simulink model "stm32f0_iap_boot"  (Simulink 7.3)
settings: Solver=ode3  SolverMode=SingleTasking  StartTime=0.0  StopTime=10.0  RelTol=1e-3
PreLoadFcn:
  | waijung.modelPreload; % Required for working with Waijung Blockset. Do not remove.
undefined symbols (not defined in the file): LQFP48, STM32F072CB
libraries: simulink x14, stm32f0_flash_lib x10, stm32f0_boot_lib x3, waijung_crc_lib x3, stm32f0_io_lib x1, stm32f0_reset_lib x1, stm32f0_device_config_lib x1
CloseFcn:
  | waijung.modelClose; % Required for working with Waijung Blockset. Do not remove.
settings Model: Creator=Nav  LastModifiedBy=Krisada
settings OptimizationCC: OptimizeModelRefInitCode=on  LifeSpan=1
settings HardwareCC: ProdEndianess=LittleEndian  ProdHWDeviceType=ARM Compatible->Cortex - M0  TargetEndianess=LittleEndian  TargetHWDeviceType=ARM Compatible->Cortex - M0
settings RTWCC: SystemTargetFile=stm32f0.tlc  GenerateMakefile=off  TemplateMakefile=ert_default_tmf  Description=STM32F0 Target  ProcessScript=stm32f0_make_rtw_hook
settings CodeAppCC: IgnoreCustomStorageClasses=off
settings STFCustomTargetCC: ModelReferenceCompliant=off  CombineOutputUpdateFcns=on  ERTCustomFileBanners=on  SupportContinuousTime=off  SupportNonInlinedSFcns=off  SystemTargetFile=stm32f0.tlc
settings ERTTargetCC: MultiwordLength=2048  ModelReferenceCompliant=off  ParMdlRefBuildCompliant=off  CompOptLevelCompliant=off  ERTFirstTimeCompliant=off  ModelStepFunctionPrototypeControlCompliant=off  CPPClassGenCompliant=off  InlinedParameterPlacement=NonHierarchical  ERTSrcFileBannerTemplate=stm32f0_code_template.cgt  ERTHdrFileBannerTemplate=stm32f0_code_template.cgt  ERTDataSrcFileTemplate=stm32f0_code_template.cgt  ERTDataHdrFileTemplate=stm32f0_code_template.cgt  ERTCustomFileTemplate=stm32f0_file_process.tlc

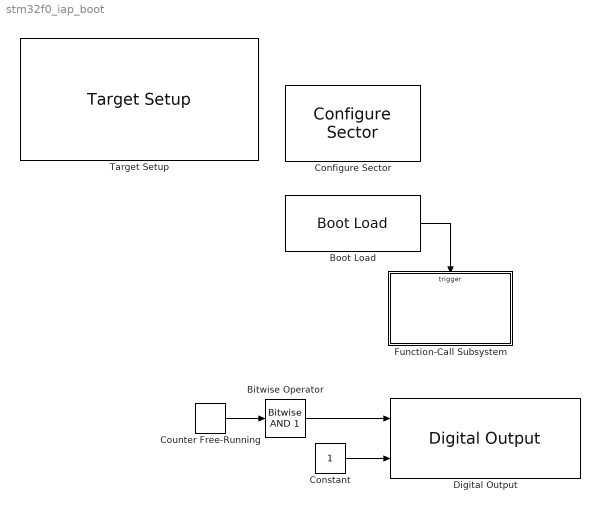
== system stm32f0_iap_boot ==
  Bitwise Operator : simulink/Logic and Bit Operations/Bitwise Operator  logicop=AND  UseBitMask=on  BitMask=1  BitMaskRealWorld=Stored Integer
  Boot Load : stm32f0_boot_lib/Boot Load  conf=Boot  flashorigin=0x8000000  flashlength=0x100000  enableisr=on  usersector=Sector 9: 0x080A0000 - 0x080BFFFF  sampletime=-1  sampletimestr=0.1  blockid=BootLoad  inputarray=[]  inputlabelarray={}  outputarray=[7]  outputlabelarray={'Call ISR'}  compat=0  confstr="[\"80A0000\",\"9\",\"8000000\"]"
  Configure Sector : stm32f0_boot_lib/Configure Sector  conf=Configure  flashorigin=0x8000000  flashlength=0x004000  enableisr=off  usersector=Sector 5: 0x08020000 - 0x0803FFFF  sampletime=-1  sampletimestr=0.1  blockid=ConfigureSector  inputarray=[]  inputlabelarray={}  outputarray=[]  outputlabelarray={}  compat=0  confstr="[\"8020000\",\"5\",\"8000000\"]"
  Constant : Constant  OutDataType=fixdt(1, 16)  OutScaling=2^0
  Counter Free-Running : simulink/Sources/Counter Free-Running  SystemSampleTime=-1  NumBits=16  tsamp=-1
  Digital Output : stm32f0_io_lib/Digital Output  use_bitband=off  port=B  speed=2  porttype=Push Pull  porttypestr=PP  use_pin0=off  use_pin1=off  use_pin2=off  use_pin3=off  use_pin4=off  use_pin5=off  use_pin6=off  use_pin7=off  use_pin8=off  use_pin9=off  use_pin10=off  use_pin11=off  use_pin12=off  use_pin13=off  use_pin14=on  use_pin15=on  pinstr=GPIO_Pin_14 | GPIO_Pin_15  usedpinarray="[0  0  0  0  0  0  0  0  0  0  0  0  0  0  1  1]"  bitbandingstr=|  sampletime=0.1  sampletimestr=0.1  blockid=DigitalOutput  enablecustomportlabel=off  cinputportlabel=In1, In2  coutputportlabel=0
      | #define DigitalOutput_B14 Peripheral_BB(GPIOB->ODR, 14)  /* Output pin */
      | #define DigitalOutput_B15 Peripheral_BB(GPIOB->ODR, 15)  /* Output pin */
  Function-Call Subsystem : Subsystem  TreatAsAtomicUnit=on
  Target Setup : stm32f0_device_config_lib/Target Setup  Priority=100  compiler=GNU ARM  previous_compiler=GNU ARM  mcu=STM32F072CB (LQFP48)  mcustr=STM32F072CB  stdlib=STM32F072  clockconfig=STM32F072B-DISCO Default (HSIOSC-8MHz/HCLK-48MHz)  system_stm32f0xx_c_path=F:\trunk\targets\stm32f0_target\stm32f0\utils\STM32F0xx_AN4055\stm32f0_default\hsi8mhz_pll_hclk48mhz  showmemoryconfiguration=off  stacksize=0x400  heapsize=0x200  enableautocompiledownload=on  fullchiperase=off  programmerinterface=aMG USB Connect  editctrlstr=on  compilercontrolstr=$(patsubst %, -I%, .) -mcpu=cortex-m0 -mthumb -mabi=aapcs -Wall -O3 -mfloat-abi=soft -ffunction-sections -fdata-sections -fno-strict-aliasing -fno-builtin --short-enums  assemblercontrolstr=$(patsubst %, -I%, .) -mcpu=cortex-m0 -mtune=cortex-m0 -mthumb -Wall -O3 -Wa,-amhls=$(<:.s=.lst) -D__STACK_SIZE=$(STACK_SIZE) -D__HEAP_SIZE=$(HEAP_SIZE)  linkercontrolstr="-T$(LD_SCRIPT) -Wl,-Map=$(MAP),--cref,--no-warn-mismatch -mcpu=cortex-m0 -mthumb  -Wall -O3 -mabi=aapcs -lc -specs=nosys.specs"  runafterdownload=on  execprofile=None  profileruart=3  profilerbaud=500000  profilertxpin=Not used  profilerinitstr=0.1,48000000,4800000,500000,0  manualsetsampletime=off  sampletime=0.1  blockid=TargetSetup  systickreloadvalue=4800000  hseval=8000000  lastprofileruart=3  hclk=48000000  flashorigin=0x8000000  flashlength=0x004000  ramorigin=0x20000000  ramlength=16k  useextram=off
  wires:
  Boot Load/1 -> Function-Call Subsystem/Trigger
  Counter Free-Running/1 -> Bitwise Operator/1
  Bitwise Operator/1 -> Digital Output/1
  Constant/1 -> Digital Output/2

== system stm32f0_iap_boot/Function-Call Subsystem ==
  note: ## Can be use to force to entering boot mode by pin
  function : TriggerPort  TriggerType=function-call
  Constant : Constant  OutDataTypeMode=uint8  OutDataType=fixdt(1, 16)  OutScaling=2^0  OutDataTypeStr=uint8
  Subsystem : Subsystem
  wires:
  Constant/1 -> Subsystem/Enable

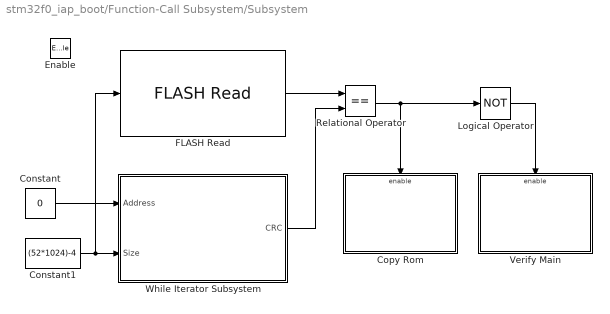
== system stm32f0_iap_boot/Function-Call Subsystem/Subsystem ==
  Enable : EnablePort
  Constant : Constant  Value=0  OutDataTypeMode=uint32  OutDataType=fixdt(1, 16)  OutScaling=2^0  OutDataTypeStr=uint32
  Constant1 : Constant  Value=(52*1024)-4  OutDataTypeMode=uint32  OutDataType=fixdt(1, 16)  OutScaling=2^0  OutDataTypeStr=uint32
  Copy Rom : Subsystem  TreatAsAtomicUnit=on
  FLASH Read : stm32f0_flash_lib/FLASH Read  conf=Read  startaddress=0x8011000  pagesize=2k  datatype=uint32  enablestatus=off  sampletime=inf  filename='stm32f0_iap_boot.flash'  enablecustomportlabel=off  cinputportlabel=0  portpinstr=0  blockid=FunctionCallSubsystemSubsystemFLASHRead  inputporttype=[7]  inputportwidth=[]  inputportlabel={'Offset'}  outputporttype=[7]  outputportwidth=[]  outputportlabel={'Data'}  compat=0  optionstring="[\"8011000\",\"0\"]"
  Logical Operator : Logic  Operator=NOT  AllPortsSameDT=off  OutDataTypeMode=boolean  LogicDataType=fixdt(0, 8)  OutDataTypeStr=boolean
  Relational Operator : RelationalOperator  Operator===  LogicOutDataTypeMode=boolean  LogicDataType=fixdt(0, 8)  OutDataTypeStr=boolean
  Verify Main : Subsystem  TreatAsAtomicUnit=on
  While Iterator Subsystem : Subsystem  TreatAsAtomicUnit=on
  wires:
  Constant/1 -> While Iterator Subsystem/1(Address)
  Constant1/1 -> While Iterator Subsystem/2(Size), FLASH Read/1
  FLASH Read/1 -> Relational Operator/1
  While Iterator Subsystem/1(CRC) -> Relational Operator/2
  Relational Operator/1 -> Copy Rom/Enable, Logical Operator/1
  Logical Operator/1 -> Verify Main/Enable

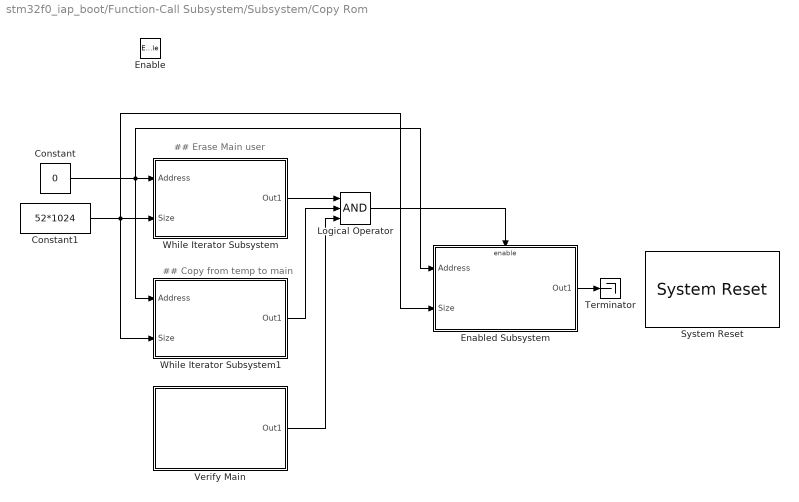
== system stm32f0_iap_boot/Function-Call Subsystem/Subsystem/Copy Rom ==
  note: ## Erase Main user
  note: ## Copy from temp to main
  Enable : EnablePort
  Constant : Constant  Value=0  OutDataTypeMode=uint32  OutDataType=fixdt(1, 16)  OutScaling=2^0  OutDataTypeStr=uint32
  Constant1 : Constant  Value=52*1024  OutDataTypeMode=uint32  OutDataType=fixdt(1, 16)  OutScaling=2^0  OutDataTypeStr=uint32
  Enabled Subsystem : Subsystem  Priority=0  TreatAsAtomicUnit=on
  Logical Operator : Logic  Inputs=3  AllPortsSameDT=off  OutDataTypeMode=boolean  LogicDataType=fixdt(0, 8)  OutDataTypeStr=boolean
  System Reset : stm32f0_reset_lib/System Reset  Priority=1  conf=<empty>  sampletime=inf  sampletimestr=-1  blockid=FunctionCallSubsystemSubsystemCopyRomSystemReset  inputarray=[]  inputlabelarray={}  outputarray=[]  outputlabelarray={}  compat=0  confstr="[\"Param1\",\"Param1\"]"
  Terminator : Terminator
  Verify Main : Subsystem  Priority=4  TreatAsAtomicUnit=on
  While Iterator Subsystem : Subsystem  Priority=2  TreatAsAtomicUnit=on
  While Iterator Subsystem1 : Subsystem  Priority=3  TreatAsAtomicUnit=on
  wires:
  Constant/1 -> While Iterator Subsystem/1(Address), While Iterator Subsystem1/1(Address), Enabled Subsystem/1(Address)
  Constant1/1 -> While Iterator Subsystem/2(Size), While Iterator Subsystem1/2(Size), Enabled Subsystem/2(Size)
  While Iterator Subsystem/1(Out1) -> Logical Operator/1
  While Iterator Subsystem1/1(Out1) -> Logical Operator/2
  Logical Operator/1 -> Enabled Subsystem/Enable
  Verify Main/1(Out1) -> Logical Operator/3
  Enabled Subsystem/1(Out1) -> Terminator/1

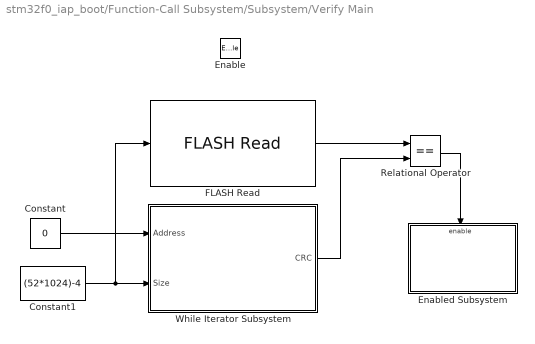
== system stm32f0_iap_boot/Function-Call Subsystem/Subsystem/Verify Main ==
  Enable : EnablePort
  Constant : Constant  Value=0  OutDataTypeMode=uint32  OutDataType=fixdt(1, 16)  OutScaling=2^0  OutDataTypeStr=uint32
  Constant1 : Constant  Value=(52*1024)-4  OutDataTypeMode=uint32  OutDataType=fixdt(1, 16)  OutScaling=2^0  OutDataTypeStr=uint32
  Enabled Subsystem : Subsystem  TreatAsAtomicUnit=on
  FLASH Read : stm32f0_flash_lib/FLASH Read  conf=Read  startaddress=0x8004000  pagesize=2k  datatype=uint32  enablestatus=off  sampletime=inf  filename='stm32f0_iap_boot.flash'  enablecustomportlabel=off  cinputportlabel=0  portpinstr=0  blockid=FunctionCallSubsystemSubsystemVerifyMainFLASHRead  inputporttype=[7]  inputportwidth=[]  inputportlabel={'Offset'}  outputporttype=[7]  outputportwidth=[]  outputportlabel={'Data'}  compat=0  optionstring="[\"8004000\",\"0\"]"
  Relational Operator : RelationalOperator  Operator===  LogicOutDataTypeMode=boolean  LogicDataType=fixdt(0, 8)  OutDataTypeStr=boolean
  While Iterator Subsystem : Subsystem  TreatAsAtomicUnit=on
  wires:
  Constant/1 -> While Iterator Subsystem/1(Address)
  Constant1/1 -> While Iterator Subsystem/2(Size), FLASH Read/1
  FLASH Read/1 -> Relational Operator/1
  While Iterator Subsystem/1(CRC) -> Relational Operator/2
  Relational Operator/1 -> Enabled Subsystem/Enable

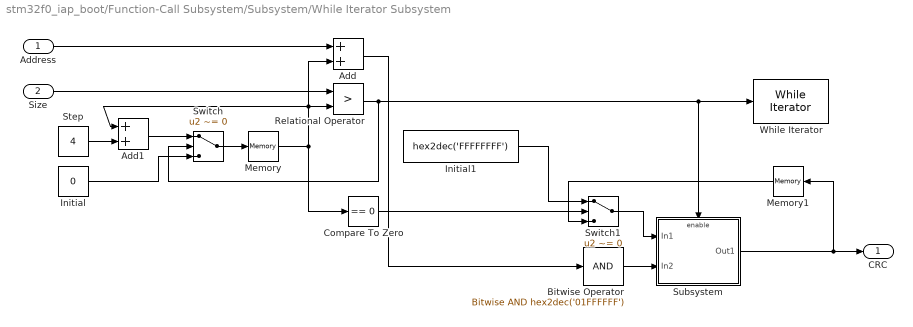
== system stm32f0_iap_boot/Function-Call Subsystem/Subsystem/While Iterator Subsystem ==
  Address : Inport  OutDataType=fixdt(1, 16)  OutScaling=2^0
  Size : Inport  Port=2  OutDataType=fixdt(1, 16)  OutScaling=2^0
  Add : Sum  OutDataType=fixdt(1, 16)  OutScaling=2^-10
  Add1 : Sum  OutDataType=fixdt(1, 16)  OutScaling=2^-10
  Bitwise Operator : simulink/Logic and Bit Operations/Bitwise Operator  logicop=AND  UseBitMask=on  BitMask=hex2dec('01FFFFFF')  BitMaskRealWorld=Stored Integer
  Compare To Zero : simulink/Logic and Bit Operations/Compare To Zero  SystemSampleTime=-1  relop===  LogicOutDataTypeMode=uint8  ZeroCross=off
  Initial : Constant  Value=0  OutDataTypeMode=uint32  OutDataType=fixdt(1, 16)  OutScaling=2^0  OutDataTypeStr=uint32
  Initial1 : Constant  Value=hex2dec('FFFFFFFF')  OutDataTypeMode=uint32  OutDataType=fixdt(1, 16)  OutScaling=2^0  OutDataTypeStr=uint32
  Memory : Memory  InheritSampleTime=on  LinearizeMemory=on
  Memory1 : Memory  InheritSampleTime=on  LinearizeMemory=on
  Relational Operator : RelationalOperator  Operator=>  LogicOutDataTypeMode=boolean  LogicDataType=fixdt(0, 8)  OutDataTypeStr=boolean
  Step : Constant  Value=4  OutDataTypeMode=uint32  OutDataType=fixdt(1, 16)  OutScaling=2^0  OutDataTypeStr=uint32
  Subsystem : Subsystem
  Switch : Switch  Criteria=u2 ~= 0  OutDataType=fixdt(1, 16)  OutScaling=2^0
  Switch1 : Switch  Criteria=u2 ~= 0  OutDataType=fixdt(1, 16)  OutScaling=2^0
  While Iterator : WhileIterator  MaxIters=-1  WhileBlockType=do-while
  CRC : Outport  OutDataType=fixdt(1, 16)  OutScaling=2^0
  wires:
  Initial/1 -> Switch/3
  Add1/1 -> Switch/1
  Relational Operator/1 -> Switch/2, While Iterator/1, Subsystem/Enable
  Switch/1 -> Memory/1
  Size/1 -> Relational Operator/1
  Step/1 -> Add1/2
  Add/1 -> Bitwise Operator/1
  Memory/1 -> Add/2, Relational Operator/2, Add1/1, Compare To Zero/1
  Address/1 -> Add/1
  Compare To Zero/1 -> Switch1/2
  Initial1/1 -> Switch1/1
  Switch1/1 -> Subsystem/1(In1)
  Subsystem/1(Out1) -> Memory1/1, CRC/1
  Memory1/1 -> Switch1/3
  Bitwise Operator/1 -> Subsystem/2(In2)

== system stm32f0_iap_boot/Function-Call Subsystem/Subsystem/Copy Rom/Enabled Subsystem ==
  Address : Inport  OutDataType=fixdt(1, 16)  OutScaling=2^0
  Size : Inport  Port=2  OutDataType=fixdt(1, 16)  OutScaling=2^0
  Enable : EnablePort
  While Iterator Subsystem : Subsystem  TreatAsAtomicUnit=on
  Out1 : Outport  OutDataType=fixdt(1, 16)  OutScaling=2^0
  wires:
  Address/1 -> While Iterator Subsystem/1(Address)
  Size/1 -> While Iterator Subsystem/2(Size)
  While Iterator Subsystem/1(Out1) -> Out1/1

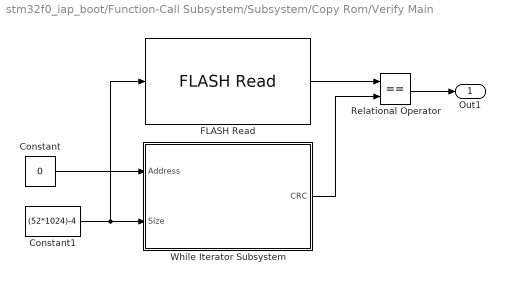
== system stm32f0_iap_boot/Function-Call Subsystem/Subsystem/Copy Rom/Verify Main ==
  Constant : Constant  Value=0  OutDataTypeMode=uint32  OutDataType=fixdt(1, 16)  OutScaling=2^0  OutDataTypeStr=uint32
  Constant1 : Constant  Value=(52*1024)-4  OutDataTypeMode=uint32  OutDataType=fixdt(1, 16)  OutScaling=2^0  OutDataTypeStr=uint32
  FLASH Read : stm32f0_flash_lib/FLASH Read  conf=Read  startaddress=0x8004000  pagesize=2k  datatype=uint32  enablestatus=off  sampletime=inf  filename='stm32f0_iap_boot.flash'  enablecustomportlabel=off  cinputportlabel=0  portpinstr=0  blockid=FunctionCallSubsystemSubsystemCopyRomVerifyMainFLASHRead  inputporttype=[7]  inputportwidth=[]  inputportlabel={'Offset'}  outputporttype=[7]  outputportwidth=[]  outputportlabel={'Data'}  compat=0  optionstring="[\"8004000\",\"0\"]"
  Relational Operator : RelationalOperator  Operator===  LogicOutDataTypeMode=boolean  LogicDataType=fixdt(0, 8)  OutDataTypeStr=boolean
  While Iterator Subsystem : Subsystem  TreatAsAtomicUnit=on
  Out1 : Outport  OutDataType=fixdt(1, 16)  OutScaling=2^0
  wires:
  While Iterator Subsystem/1(CRC) -> Relational Operator/2
  FLASH Read/1 -> Relational Operator/1
  Constant1/1 -> FLASH Read/1, While Iterator Subsystem/2(Size)
  Constant/1 -> While Iterator Subsystem/1(Address)
  Relational Operator/1 -> Out1/1

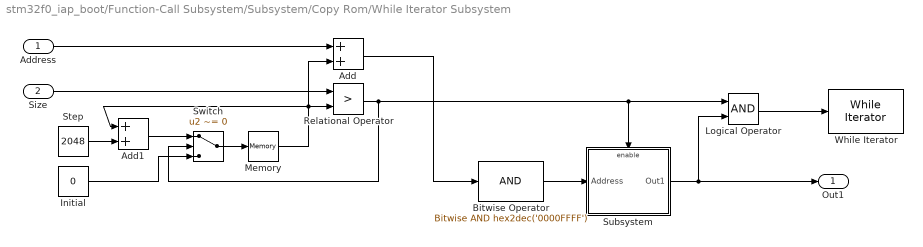
== system stm32f0_iap_boot/Function-Call Subsystem/Subsystem/Copy Rom/While Iterator Subsystem ==
  Address : Inport  OutDataType=fixdt(1, 16)  OutScaling=2^0
  Size : Inport  Port=2  OutDataType=fixdt(1, 16)  OutScaling=2^0
  Add : Sum  OutDataType=fixdt(1, 16)  OutScaling=2^-10
  Add1 : Sum  OutDataType=fixdt(1, 16)  OutScaling=2^-10
  Bitwise Operator : simulink/Logic and Bit Operations/Bitwise Operator  logicop=AND  UseBitMask=on  BitMask=hex2dec('0000FFFF')  BitMaskRealWorld=Stored Integer
  Initial : Constant  Value=0  OutDataTypeMode=uint32  OutDataType=fixdt(1, 16)  OutScaling=2^0  OutDataTypeStr=uint32
  Logical Operator : Logic  AllPortsSameDT=off  OutDataTypeMode=boolean  LogicDataType=fixdt(0, 8)  OutDataTypeStr=boolean
  Memory : Memory  InheritSampleTime=on  LinearizeMemory=on
  Relational Operator : RelationalOperator  Operator=>  LogicOutDataTypeMode=boolean  LogicDataType=fixdt(0, 8)  OutDataTypeStr=boolean
  Step : Constant  Value=2048  OutDataTypeMode=uint32  OutDataType=fixdt(1, 16)  OutScaling=2^0  OutDataTypeStr=uint32
  Subsystem : Subsystem
  Switch : Switch  Criteria=u2 ~= 0  OutDataType=fixdt(1, 16)  OutScaling=2^0
  While Iterator : WhileIterator  MaxIters=-1  WhileBlockType=do-while
  Out1 : Outport  OutDataType=fixdt(1, 16)  OutScaling=2^0
  wires:
  Initial/1 -> Switch/3
  Add1/1 -> Switch/1
  Relational Operator/1 -> Switch/2, Subsystem/Enable, Logical Operator/1
  Switch/1 -> Memory/1
  Size/1 -> Relational Operator/1
  Step/1 -> Add1/2
  Add/1 -> Bitwise Operator/1
  Memory/1 -> Add/2, Relational Operator/2, Add1/1
  Address/1 -> Add/1
  Bitwise Operator/1 -> Subsystem/1(Address)
  Subsystem/1(Out1) -> Out1/1, Logical Operator/2
  Logical Operator/1 -> While Iterator/1

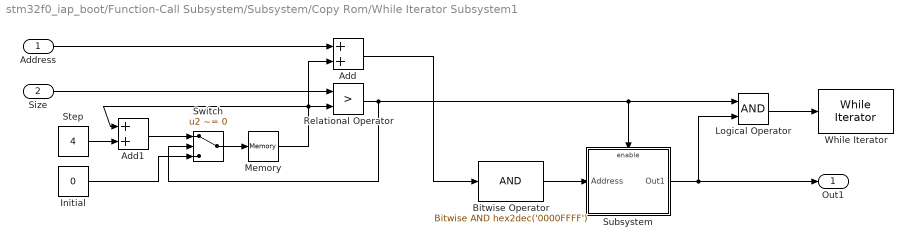
== system stm32f0_iap_boot/Function-Call Subsystem/Subsystem/Copy Rom/While Iterator Subsystem1 ==
  Address : Inport  OutDataType=fixdt(1, 16)  OutScaling=2^0
  Size : Inport  Port=2  OutDataType=fixdt(1, 16)  OutScaling=2^0
  Add : Sum  OutDataType=fixdt(1, 16)  OutScaling=2^-10
  Add1 : Sum  OutDataType=fixdt(1, 16)  OutScaling=2^-10
  Bitwise Operator : simulink/Logic and Bit Operations/Bitwise Operator  logicop=AND  UseBitMask=on  BitMask=hex2dec('0000FFFF')  BitMaskRealWorld=Stored Integer
  Initial : Constant  Value=0  OutDataTypeMode=uint32  OutDataType=fixdt(1, 16)  OutScaling=2^0  OutDataTypeStr=uint32
  Logical Operator : Logic  AllPortsSameDT=off  OutDataTypeMode=boolean  LogicDataType=fixdt(0, 8)  OutDataTypeStr=boolean
  Memory : Memory  InheritSampleTime=on  LinearizeMemory=on
  Relational Operator : RelationalOperator  Operator=>  LogicOutDataTypeMode=boolean  LogicDataType=fixdt(0, 8)  OutDataTypeStr=boolean
  Step : Constant  Value=4  OutDataTypeMode=uint32  OutDataType=fixdt(1, 16)  OutScaling=2^0  OutDataTypeStr=uint32
  Subsystem : Subsystem
  Switch : Switch  Criteria=u2 ~= 0  OutDataType=fixdt(1, 16)  OutScaling=2^0
  While Iterator : WhileIterator  MaxIters=-1  WhileBlockType=do-while
  Out1 : Outport  OutDataType=fixdt(1, 16)  OutScaling=2^0
  wires:
  Bitwise Operator/1 -> Subsystem/1(Address)
  Address/1 -> Add/1
  Memory/1 -> Add1/1, Relational Operator/2, Add/2
  Add/1 -> Bitwise Operator/1
  Step/1 -> Add1/2
  Size/1 -> Relational Operator/1
  Switch/1 -> Memory/1
  Relational Operator/1 -> Switch/2, Subsystem/Enable, Logical Operator/1
  Add1/1 -> Switch/1
  Initial/1 -> Switch/3
  Subsystem/1(Out1) -> Logical Operator/2, Out1/1
  Logical Operator/1 -> While Iterator/1

== system stm32f0_iap_boot/Function-Call Subsystem/Subsystem/Verify Main/Enabled Subsystem ==
  Enable : EnablePort
  Jump Sector : stm32f0_boot_lib/Jump Sector  conf=Goto  flashorigin=0x8000000  flashlength=0x100000  enableisr=off  usersector=Sector 8: 0x8004000 - 0x80047FF  sampletime=inf  sampletimestr=-1  blockid=FunctionCallSubsystemSubsystemVerifyMainEnabledSubsystemJumpSector  inputarray=[]  inputlabelarray={}  outputarray=[]  outputlabelarray={}  compat=0  confstr="[\"8004000\",\"8\",\"8000000\"]"

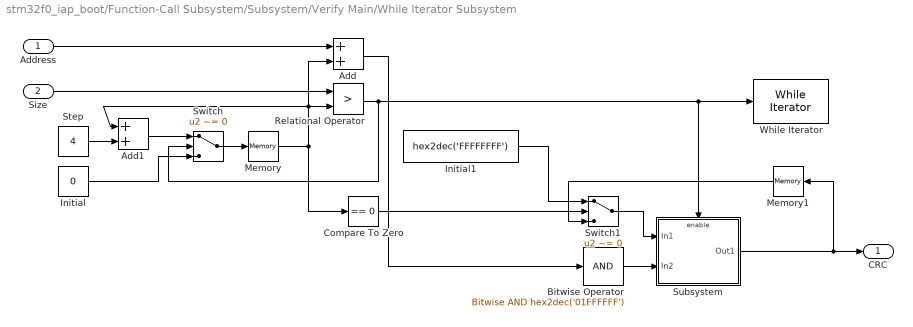
== system stm32f0_iap_boot/Function-Call Subsystem/Subsystem/Verify Main/While Iterator Subsystem ==
  Address : Inport  OutDataType=fixdt(1, 16)  OutScaling=2^0
  Size : Inport  Port=2  OutDataType=fixdt(1, 16)  OutScaling=2^0
  Add : Sum  OutDataType=fixdt(1, 16)  OutScaling=2^-10
  Add1 : Sum  OutDataType=fixdt(1, 16)  OutScaling=2^-10
  Bitwise Operator : simulink/Logic and Bit Operations/Bitwise Operator  logicop=AND  UseBitMask=on  BitMask=hex2dec('01FFFFFF')  BitMaskRealWorld=Stored Integer
  Compare To Zero : simulink/Logic and Bit Operations/Compare To Zero  SystemSampleTime=-1  relop===  LogicOutDataTypeMode=uint8  ZeroCross=off
  Initial : Constant  Value=0  OutDataTypeMode=uint32  OutDataType=fixdt(1, 16)  OutScaling=2^0  OutDataTypeStr=uint32
  Initial1 : Constant  Value=hex2dec('FFFFFFFF')  OutDataTypeMode=uint32  OutDataType=fixdt(1, 16)  OutScaling=2^0  OutDataTypeStr=uint32
  Memory : Memory  InheritSampleTime=on  LinearizeMemory=on
  Memory1 : Memory  InheritSampleTime=on  LinearizeMemory=on
  Relational Operator : RelationalOperator  Operator=>  LogicOutDataTypeMode=boolean  LogicDataType=fixdt(0, 8)  OutDataTypeStr=boolean
  Step : Constant  Value=4  OutDataTypeMode=uint32  OutDataType=fixdt(1, 16)  OutScaling=2^0  OutDataTypeStr=uint32
  Subsystem : Subsystem
  Switch : Switch  Criteria=u2 ~= 0  OutDataType=fixdt(1, 16)  OutScaling=2^0
  Switch1 : Switch  Criteria=u2 ~= 0  OutDataType=fixdt(1, 16)  OutScaling=2^0
  While Iterator : WhileIterator  MaxIters=-1  WhileBlockType=do-while
  CRC : Outport  OutDataType=fixdt(1, 16)  OutScaling=2^0
  wires:
  Initial/1 -> Switch/3
  Add1/1 -> Switch/1
  Relational Operator/1 -> Switch/2, While Iterator/1, Subsystem/Enable
  Switch/1 -> Memory/1
  Size/1 -> Relational Operator/1
  Step/1 -> Add1/2
  Add/1 -> Bitwise Operator/1
  Memory/1 -> Add/2, Relational Operator/2, Add1/1, Compare To Zero/1
  Address/1 -> Add/1
  Compare To Zero/1 -> Switch1/2
  Initial1/1 -> Switch1/1
  Switch1/1 -> Subsystem/1(In1)
  Subsystem/1(Out1) -> Memory1/1, CRC/1
  Memory1/1 -> Switch1/3
  Bitwise Operator/1 -> Subsystem/2(In2)

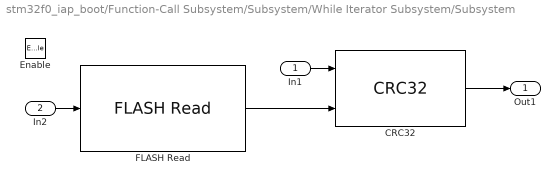
== system stm32f0_iap_boot/Function-Call Subsystem/Subsystem/While Iterator Subsystem/Subsystem ==
  In1 : Inport
  In2 : Inport  Port=2
  Enable : EnablePort
  CRC32 : waijung_crc_lib/CRC32  conf=<empty>  sampletime=-1  enablecustomportlabel=off  cinputportlabel=0  portpinstr=0  blockid=FunctionCallSubsystemSubsystemWhileIteratorSubsystemSubsystemCRC32  inputporttype=[7 7]  inputportwidth=[1 -1]  inputportlabel={'Initial','Value'}  outputporttype=[7]  outputportwidth=[]  outputportlabel={'Output'}  compat=0  optionstring="[\"Param1\",\"Param1\"]"
  FLASH Read : stm32f0_flash_lib/FLASH Read  conf=Read  startaddress=0x8011000  pagesize=2k  datatype=uint32  enablestatus=off  sampletime=inf  filename='stm32f0_iap_boot.flash'  enablecustomportlabel=off  cinputportlabel=0  portpinstr=0  blockid=FunctionCallSubsystemSubsystemWhileIteratorSubsystemSubsystemFLASHRead  inputporttype=[7]  inputportwidth=[]  inputportlabel={'Offset'}  outputporttype=[7]  outputportwidth=[]  outputportlabel={'Data'}  compat=0  optionstring="[\"8011000\",\"0\"]"
  Out1 : Outport
  wires:
  FLASH Read/1 -> CRC32/2
  In1/1 -> CRC32/1
  CRC32/1 -> Out1/1
  In2/1 -> FLASH Read/1

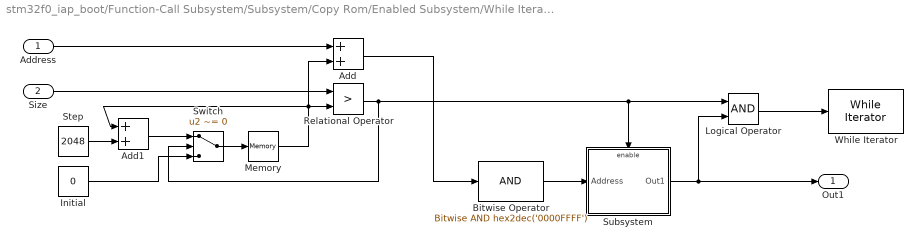
== system stm32f0_iap_boot/Function-Call Subsystem/Subsystem/Copy Rom/Enabled Subsystem/While Iterator Subsystem ==
  Address : Inport  OutDataType=fixdt(1, 16)  OutScaling=2^0
  Size : Inport  Port=2  OutDataType=fixdt(1, 16)  OutScaling=2^0
  Add : Sum  OutDataType=fixdt(1, 16)  OutScaling=2^-10
  Add1 : Sum  OutDataType=fixdt(1, 16)  OutScaling=2^-10
  Bitwise Operator : simulink/Logic and Bit Operations/Bitwise Operator  logicop=AND  UseBitMask=on  BitMask=hex2dec('0000FFFF')  BitMaskRealWorld=Stored Integer
  Initial : Constant  Value=0  OutDataTypeMode=uint32  OutDataType=fixdt(1, 16)  OutScaling=2^0  OutDataTypeStr=uint32
  Logical Operator : Logic  AllPortsSameDT=off  OutDataTypeMode=boolean  LogicDataType=fixdt(0, 8)  OutDataTypeStr=boolean
  Memory : Memory  InheritSampleTime=on  LinearizeMemory=on
  Relational Operator : RelationalOperator  Operator=>  LogicOutDataTypeMode=boolean  LogicDataType=fixdt(0, 8)  OutDataTypeStr=boolean
  Step : Constant  Value=2048  OutDataTypeMode=uint32  OutDataType=fixdt(1, 16)  OutScaling=2^0  OutDataTypeStr=uint32
  Subsystem : Subsystem
  Switch : Switch  Criteria=u2 ~= 0  OutDataType=fixdt(1, 16)  OutScaling=2^0
  While Iterator : WhileIterator  MaxIters=-1  WhileBlockType=do-while
  Out1 : Outport  OutDataType=fixdt(1, 16)  OutScaling=2^0
  wires:
  Initial/1 -> Switch/3
  Add1/1 -> Switch/1
  Relational Operator/1 -> Switch/2, Subsystem/Enable, Logical Operator/1
  Switch/1 -> Memory/1
  Size/1 -> Relational Operator/1
  Step/1 -> Add1/2
  Add/1 -> Bitwise Operator/1
  Memory/1 -> Add/2, Relational Operator/2, Add1/1
  Address/1 -> Add/1
  Bitwise Operator/1 -> Subsystem/1(Address)
  Subsystem/1(Out1) -> Out1/1, Logical Operator/2
  Logical Operator/1 -> While Iterator/1

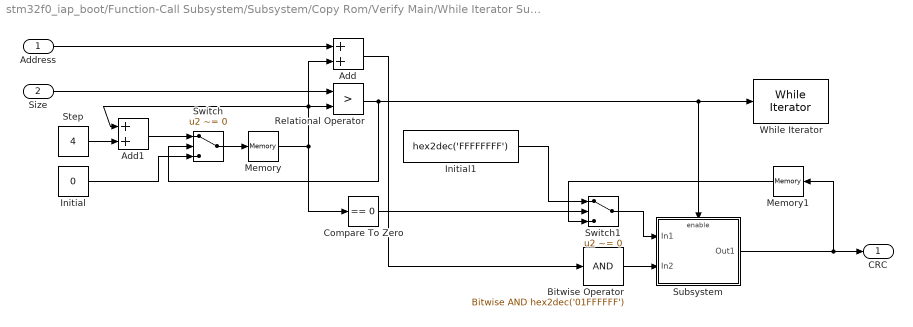
== system stm32f0_iap_boot/Function-Call Subsystem/Subsystem/Copy Rom/Verify Main/While Iterator Subsystem ==
  Address : Inport  OutDataType=fixdt(1, 16)  OutScaling=2^0
  Size : Inport  Port=2  OutDataType=fixdt(1, 16)  OutScaling=2^0
  Add : Sum  OutDataType=fixdt(1, 16)  OutScaling=2^-10
  Add1 : Sum  OutDataType=fixdt(1, 16)  OutScaling=2^-10
  Bitwise Operator : simulink/Logic and Bit Operations/Bitwise Operator  logicop=AND  UseBitMask=on  BitMask=hex2dec('01FFFFFF')  BitMaskRealWorld=Stored Integer
  Compare To Zero : simulink/Logic and Bit Operations/Compare To Zero  SystemSampleTime=-1  relop===  LogicOutDataTypeMode=uint8  ZeroCross=off
  Initial : Constant  Value=0  OutDataTypeMode=uint32  OutDataType=fixdt(1, 16)  OutScaling=2^0  OutDataTypeStr=uint32
  Initial1 : Constant  Value=hex2dec('FFFFFFFF')  OutDataTypeMode=uint32  OutDataType=fixdt(1, 16)  OutScaling=2^0  OutDataTypeStr=uint32
  Memory : Memory  InheritSampleTime=on  LinearizeMemory=on
  Memory1 : Memory  InheritSampleTime=on  LinearizeMemory=on
  Relational Operator : RelationalOperator  Operator=>  LogicOutDataTypeMode=boolean  LogicDataType=fixdt(0, 8)  OutDataTypeStr=boolean
  Step : Constant  Value=4  OutDataTypeMode=uint32  OutDataType=fixdt(1, 16)  OutScaling=2^0  OutDataTypeStr=uint32
  Subsystem : Subsystem
  Switch : Switch  Criteria=u2 ~= 0  OutDataType=fixdt(1, 16)  OutScaling=2^0
  Switch1 : Switch  Criteria=u2 ~= 0  OutDataType=fixdt(1, 16)  OutScaling=2^0
  While Iterator : WhileIterator  MaxIters=-1  WhileBlockType=do-while
  CRC : Outport  OutDataType=fixdt(1, 16)  OutScaling=2^0
  wires:
  Bitwise Operator/1 -> Subsystem/2(In2)
  Memory1/1 -> Switch1/3
  Subsystem/1(Out1) -> CRC/1, Memory1/1
  Switch1/1 -> Subsystem/1(In1)
  Initial1/1 -> Switch1/1
  Compare To Zero/1 -> Switch1/2
  Address/1 -> Add/1
  Memory/1 -> Compare To Zero/1, Add1/1, Relational Operator/2, Add/2
  Add/1 -> Bitwise Operator/1
  Step/1 -> Add1/2
  Size/1 -> Relational Operator/1
  Switch/1 -> Memory/1
  Relational Operator/1 -> Subsystem/Enable, While Iterator/1, Switch/2
  Add1/1 -> Switch/1
  Initial/1 -> Switch/3

== system stm32f0_iap_boot/Function-Call Subsystem/Subsystem/Copy Rom/While Iterator Subsystem/Subsystem ==
  Address : Inport
  Enable : EnablePort
  Compare To Constant : simulink/Logic and Bit Operations/Compare To Constant  SystemSampleTime=-1  relop===  const=4  LogicOutDataTypeMode=uint8  ZeroCross=off
  FLASH Erase : stm32f0_flash_lib/FLASH Erase  conf=Erase  startaddress=0x8004000  pagesize=2k  datatype=int32  enablestatus=on  sampletime=inf  filename='stm32f0_iap_boot.flash'  enablecustomportlabel=off  cinputportlabel=0  portpinstr=0  blockid=FunctionCallSubsystemSubsystemCopyRomWhileIteratorSubsystemSubsystemFLASHErase  inputporttype=[7]  inputportwidth=[]  inputportlabel={'Page Offset'}  outputporttype=[3]  outputportwidth=[]  outputportlabel={'Status'}  compat=0  optionstring="[\"8004000\",\"0\"]"
  Out1 : Outport  OutDataType=fixdt(1, 16)  OutScaling=2^0
  wires:
  Address/1 -> FLASH Erase/1
  FLASH Erase/1 -> Compare To Constant/1
  Compare To Constant/1 -> Out1/1

== system stm32f0_iap_boot/Function-Call Subsystem/Subsystem/Copy Rom/While Iterator Subsystem1/Subsystem ==
  Address : Inport
  Enable : EnablePort
  Compare To Constant : simulink/Logic and Bit Operations/Compare To Constant  SystemSampleTime=-1  relop===  const=4  LogicOutDataTypeMode=uint8  ZeroCross=off
  FLASH Read : stm32f0_flash_lib/FLASH Read  conf=Read  startaddress=0x8011000  pagesize=2k  datatype=uint32  enablestatus=off  sampletime=inf  filename='stm32f0_iap_boot.flash'  enablecustomportlabel=off  cinputportlabel=0  portpinstr=0  blockid=FunctionCallSubsystemSubsystemCopyRomWhileIteratorSubsystem1SubsystemFLASHRead  inputporttype=[7]  inputportwidth=[]  inputportlabel={'Offset'}  outputporttype=[7]  outputportwidth=[]  outputportlabel={'Data'}  compat=0  optionstring="[\"8011000\",\"0\"]"
  FLASH Write : stm32f0_flash_lib/FLASH Write  conf=Write  startaddress=0x8004000  pagesize=2k  datatype=uint32  enablestatus=on  sampletime=inf  filename='stm32f0_iap_boot.flash'  enablecustomportlabel=off  cinputportlabel=0  portpinstr=0  blockid=FunctionCallSubsystemSubsystemCopyRomWhileIteratorSubsystem1SubsystemFLASHWrite  inputporttype=[7 7]  inputportwidth=[]  inputportlabel={'Offset','Data (uint32)'}  outputporttype=[3]  outputportwidth=[]  outputportlabel={'Status'}  compat=0  optionstring="[\"8004000\",\"0\"]"
  Out1 : Outport  OutDataType=fixdt(1, 16)  OutScaling=2^0
  wires:
  Address/1 -> FLASH Read/1, FLASH Write/1
  FLASH Read/1 -> FLASH Write/2
  FLASH Write/1 -> Compare To Constant/1
  Compare To Constant/1 -> Out1/1

== system stm32f0_iap_boot/Function-Call Subsystem/Subsystem/Verify Main/While Iterator Subsystem/Subsystem ==
  In1 : Inport
  In2 : Inport  Port=2
  Enable : EnablePort
  CRC32 : waijung_crc_lib/CRC32  conf=<empty>  sampletime=-1  enablecustomportlabel=off  cinputportlabel=0  portpinstr=0  blockid=FunctionCallSubsystemSubsystemVerifyMainWhileIteratorSubsystemSubsystemCRC32  inputporttype=[7 7]  inputportwidth=[1 -1]  inputportlabel={'Initial','Value'}  outputporttype=[7]  outputportwidth=[]  outputportlabel={'Output'}  compat=0  optionstring="[\"Param1\",\"Param1\"]"
  FLASH Read : stm32f0_flash_lib/FLASH Read  conf=Read  startaddress=0x8004000  pagesize=2k  datatype=uint32  enablestatus=off  sampletime=inf  filename='stm32f0_iap_boot.flash'  enablecustomportlabel=off  cinputportlabel=0  portpinstr=0  blockid=FunctionCallSubsystemSubsystemVerifyMainWhileIteratorSubsystemSubsystemFLASHRead  inputporttype=[7]  inputportwidth=[]  inputportlabel={'Offset'}  outputporttype=[7]  outputportwidth=[]  outputportlabel={'Data'}  compat=0  optionstring="[\"8004000\",\"0\"]"
  Out1 : Outport
  wires:
  FLASH Read/1 -> CRC32/2
  In1/1 -> CRC32/1
  CRC32/1 -> Out1/1
  In2/1 -> FLASH Read/1

== system stm32f0_iap_boot/Function-Call Subsystem/Subsystem/Copy Rom/Enabled Subsystem/While Iterator Subsystem/Subsystem ==
  Address : Inport
  Enable : EnablePort
  Compare To Constant : simulink/Logic and Bit Operations/Compare To Constant  SystemSampleTime=-1  relop===  const=4  LogicOutDataTypeMode=uint8  ZeroCross=off
  FLASH Erase : stm32f0_flash_lib/FLASH Erase  conf=Erase  startaddress=0x8011000  pagesize=2k  datatype=int32  enablestatus=on  sampletime=inf  filename='stm32f0_iap_boot.flash'  enablecustomportlabel=off  cinputportlabel=0  portpinstr=0  blockid=FunctionCallSubsystemSubsystemCopyRomEnabledSubsystemWhileIteratorSubsystemSubsystemFLASHErase  inputporttype=[7]  inputportwidth=[]  inputportlabel={'Page Offset'}  outputporttype=[3]  outputportwidth=[]  outputportlabel={'Status'}  compat=0  optionstring="[\"8011000\",\"0\"]"
  Out1 : Outport  OutDataType=fixdt(1, 16)  OutScaling=2^0
  wires:
  Address/1 -> FLASH Erase/1
  FLASH Erase/1 -> Compare To Constant/1
  Compare To Constant/1 -> Out1/1

== system stm32f0_iap_boot/Function-Call Subsystem/Subsystem/Copy Rom/Verify Main/While Iterator Subsystem/Subsystem ==
  In1 : Inport
  In2 : Inport  Port=2
  Enable : EnablePort
  CRC32 : waijung_crc_lib/CRC32  conf=<empty>  sampletime=-1  enablecustomportlabel=off  cinputportlabel=0  portpinstr=0  blockid=FunctionCallSubsystemSubsystemCopyRomVerifyMainWhileIteratorSubsystemSubsystemCRC32  inputporttype=[7 7]  inputportwidth=[1 -1]  inputportlabel={'Initial','Value'}  outputporttype=[7]  outputportwidth=[]  outputportlabel={'Output'}  compat=0  optionstring="[\"Param1\",\"Param1\"]"
  FLASH Read : stm32f0_flash_lib/FLASH Read  conf=Read  startaddress=0x8004000  pagesize=2k  datatype=uint32  enablestatus=off  sampletime=inf  filename='stm32f0_iap_boot.flash'  enablecustomportlabel=off  cinputportlabel=0  portpinstr=0  blockid=FunctionCallSubsystemSubsystemCopyRomVerifyMainWhileIteratorSubsystemSubsystemFLASHRead  inputporttype=[7]  inputportwidth=[]  inputportlabel={'Offset'}  outputporttype=[7]  outputportwidth=[]  outputportlabel={'Data'}  compat=0  optionstring="[\"8004000\",\"0\"]"
  Out1 : Outport
  wires:
  In2/1 -> FLASH Read/1
  CRC32/1 -> Out1/1
  In1/1 -> CRC32/1
  FLASH Read/1 -> CRC32/2
